simulink model "gm_gm_decoderN4ByFullMatlabOneFunction"  (R2016b)
settings: Solver=FixedStepDiscrete  StartTime=0.0  StopTime=10.0  RelTol=1e-3
settings Model: Creator=hasee  LastModifiedBy=hasee
settings DataIOCC: LimitDataPoints=on  SaveOutput=off  SaveTime=off
settings OptimizationCC: BlockReduction=off  ConditionallyExecuteInputs=off  DefaultParameterBehavior=Inlined  LifeSpan=inf
settings DebuggingCC: AlgebraicLoopMsg=error  InheritedTsInSrcMsg=none  SingleTaskRateTransMsg=error  AllowSymbolicDim=off  StrictBusMsg=ErrorOnBusTreatedAsVector  SFUnexpectedBacktrackingDiag=warning  SFNoUnconditionalDefaultTransitionDiag=warning  SFExecutionAtInitializationDiag=none
settings HardwareCC: ProdBitPerPointer=32  ProdBitPerSizeT=32  ProdBitPerPtrDiffT=32  ProdLargestAtomicFloat=None  ProdIntDivRoundTo=Undefined  ProdEndianess=Unspecified  ProdWordSize=32  ProdHWDeviceType=ASIC/FPGA->ASIC/FPGA  ProdEqTarget=off
settings GRTTargetCC: TargetLangStandard=C89/C90 (ANSI)  GeneratePreprocessorConditionals=Disable all
settings ConfigComp: CovScope=ReferencedModels  CovMetricSettings=dw  CovHtmlReporting=on  CovSaveCumulativeToWorkspaceVar=on  CovSaveSingleToWorkspaceVar=on  CovExternalEMLEnable=off  CovSFcnEnable=off

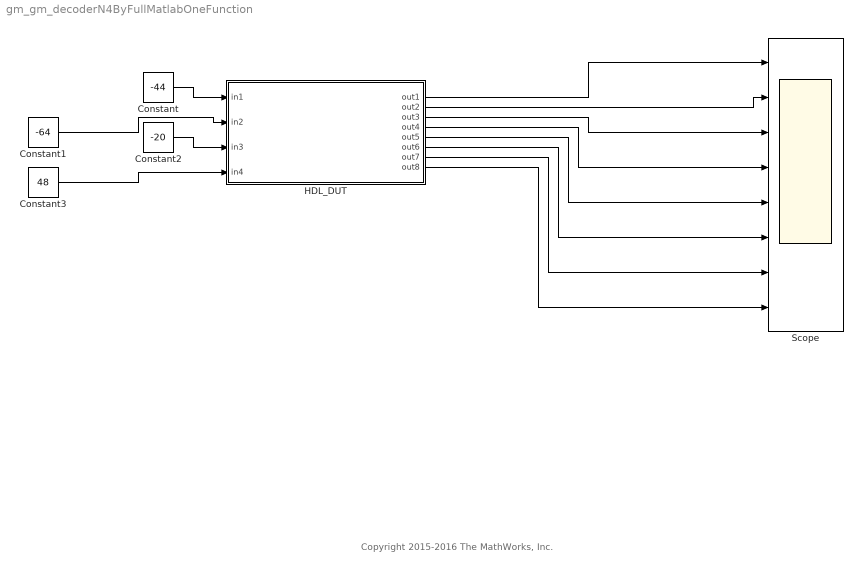
== system gm_gm_decoderN4ByFullMatlabOneFunction ==
  note: Copyright 2015-2016 The MathWorks, Inc.
  Constant : Constant  Value=-44  OutDataTypeStr=int8  SampleTime=-1
  Constant1 : Constant  Value=-64  OutDataTypeStr=int8  SampleTime=-1
  Constant2 : Constant  Value=-20  OutDataTypeStr=int8  SampleTime=-1
  Constant3 : Constant  Value=48  OutDataTypeStr=int8  SampleTime=-1
  HDL_DUT : Subsystem
  Scope : Scope  NumInputPorts=8
  wires:
  Constant/1 -> HDL_DUT/1(in1)
  Constant1/1 -> HDL_DUT/2(in2)
  Constant2/1 -> HDL_DUT/3(in3)
  Constant3/1 -> HDL_DUT/4(in4)
  HDL_DUT/1(out1) -> Scope/1
  HDL_DUT/2(out2) -> Scope/2
  HDL_DUT/3(out3) -> Scope/3
  HDL_DUT/4(out4) -> Scope/4
  HDL_DUT/5(out5) -> Scope/5
  HDL_DUT/6(out6) -> Scope/6
  HDL_DUT/7(out7) -> Scope/7
  HDL_DUT/8(out8) -> Scope/8

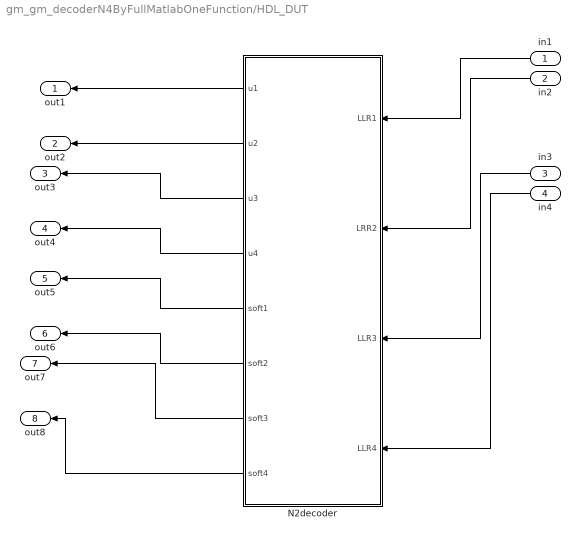
== system gm_gm_decoderN4ByFullMatlabOneFunction/HDL_DUT ==
  in1 : Inport  SampleTime=0.2
  in2 : Inport  Port=2  SampleTime=0.2
  in3 : Inport  Port=3  SampleTime=0.2
  in4 : Inport  Port=4  SampleTime=0.2
  N2decoder : Subsystem
  out1 : Outport
  out2 : Outport  Port=2
  out3 : Outport  Port=3
  out4 : Outport  Port=4
  out5 : Outport  Port=5
  out6 : Outport  Port=6
  out7 : Outport  Port=7
  out8 : Outport  Port=8
  wires:
  in1/1 -> N2decoder/1(LLR1)
  in2/1 -> N2decoder/2(LRR2)
  in3/1 -> N2decoder/3(LLR3)
  in4/1 -> N2decoder/4(LLR4)
  N2decoder/1(u1) -> out1/1
  N2decoder/2(u2) -> out2/1
  N2decoder/3(u3) -> out3/1
  N2decoder/4(u4) -> out4/1
  N2decoder/5(soft1) -> out5/1
  N2decoder/6(soft2) -> out6/1
  N2decoder/7(soft3) -> out7/1
  N2decoder/8(soft4) -> out8/1

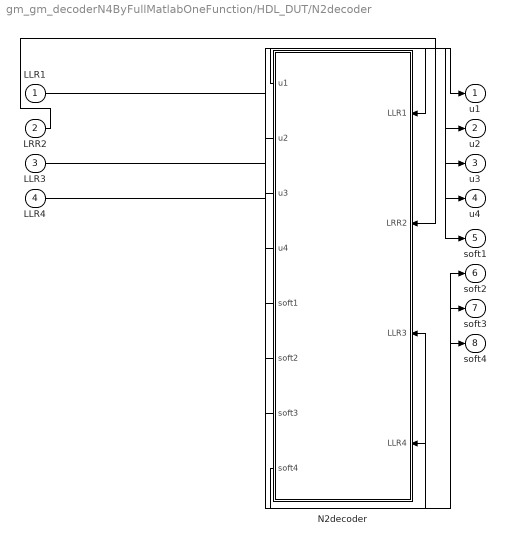
== system gm_gm_decoderN4ByFullMatlabOneFunction/HDL_DUT/N2decoder ==
  LLR1 : Inport  SampleTime=0.2
  LRR2 : Inport  Port=2  SampleTime=0.2
  LLR3 : Inport  Port=3  SampleTime=0.2
  LLR4 : Inport  Port=4  SampleTime=0.2
  N2decoder : MATLAB Function  TreatAsAtomicUnit=on
  u1 : Outport
  u2 : Outport  Port=2
  u3 : Outport  Port=3
  u4 : Outport  Port=4
  soft1 : Outport  Port=5
  soft2 : Outport  Port=6
  soft3 : Outport  Port=7
  soft4 : Outport  Port=8
  wires:
  LLR1/1 -> N2decoder/1(LLR1)
  LRR2/1 -> N2decoder/2(LRR2)
  LLR3/1 -> N2decoder/3(LLR3)
  LLR4/1 -> N2decoder/4(LLR4)
  N2decoder/1(u1) -> u1/1
  N2decoder/2(u2) -> u2/1
  N2decoder/3(u3) -> u3/1
  N2decoder/4(u4) -> u4/1
  N2decoder/5(soft1) -> soft1/1
  N2decoder/6(soft2) -> soft2/1
  N2decoder/7(soft3) -> soft3/1
  N2decoder/8(soft4) -> soft4/1

== matlab function gm_gm_decoderN4ByFullMatlabOneFunction/HDL_DUT/N2decoder/N2decoder ==
  data: LLR1 input int8; u1 output; LRR2 input int8; LLR3 input int8; LLR4 input int8; u2 output; u3 output; u4 output; soft1 output; soft2 output; soft3 output; soft4 output
function [u1,u2,u3,u4,soft1,soft2,soft3,soft4] = fcn(LLR1, LRR2, LLR3, LLR4)
%#codegen
L21y12=f(LLR1,LRR2);
L21y34=f(LLR3,LLR4);
L41y14=f(L21y12,L21y34);
soft1=L41y14;
u1=decide(soft1,1);

%计算u2
L42y14u11=g(L21y12,L21y34,u1);
soft2=L42y14u11;
u2=decide(soft2,2);

%计算u3
L22y12u12=g(LLR1,LRR2,xor(u1,u2));
L22y34u2 = g(LLR3,LLR4,u2);
L43y14u12=f(L22y12u12,L22y34u2);
soft3=L43y14u12;
u3=decide(soft3,3);

%计算u4
L44y14u13 = g(L22y12u12,L22y34u2,u3);
soft4=L44y14u13;
u4=decide(soft4,4);




%FZlookup是冻结比特位置信息，false代表这一位是冻结比特
function out = decide(soft,position)
persistent FZlookup;
if isempty(FZlookup)
    FZlookup = [false;true;true;true];
end
if FZlookup(position) == true
    if soft > 0  %PCparams.LLR(1) 就是根据最左边的LLR硬裁决
        out = false;
    else
        out = true;
    end
else
    out =FZlookup(position);
end

function out = f(in1,in2)
if (in1>0 && in2>0) ||(in1<0 && in2<0)
    out=min(abs(in1),abs(in2));
else
    out=-min(abs(in1),abs(in2));
end


function out = g(in1,in2,b)
if (b == 0)
    out=int32(in1) + int32(in2);
else
    out=int32(-in1) + int32(in2);
end

%寄存器
function y = reg(u)
% Unit delay implementation that maps to a register in hardware

persistent u_d;
if isempty(u_d)
    % defines initial value driven by unit delay at time step 0
    u_d = cast(0, 'like', u);
end

% return delayed input from last sample time hit
y = u_d;

% store the current input
u_d = u;
